simulink model "DriverSwRequest"  (R2023a)
settings: Solver=FixedStepDiscrete  StartTime=0.0  StopTime=10.0  FixedStep=0.01  RelTol=1e-3
undefined symbols (not defined in the file): reqMode
libraries: simulink x20
settings Model: RequirementInfo={} %GIDa_1a0f7f75_7b2a_416a_8409_7d146d7c864c  DataDictionary=crs_controllerdic.sldd  EnableAccessToBaseWorkspace=off  Creator=The MathWorks, Inc.  LastModifiedBy=shayashi
settings SolverCC: AlgebraicLoopSolver=TrustRegion
settings DataIOCC: SaveOutput=off  SignalLogging=off  DSMLogging=off  SaveTime=off  ReturnWorkspaceOutputs=off
settings OptimizationCC: DefaultParameterBehavior=Inlined  PassReuseOutputArgsAs=Individual arguments  EfficientTunableParamExpr=on
settings DebuggingCC: ParameterTunabilityLossMsg=error  UnconnectedInputMsg=warning  UnconnectedOutputMsg=warning  UnconnectedLineMsg=warning  ArithmeticOperatorsInVariantConditions=warning
settings ModelReferenceCC: EnableRefExpFcnMdlSchedulingChecks=on
settings SFSimCC: SimUseLocalCustomCode=off  CustomCodeUndefinedFunction=UseInterfaceOnly
settings RTWCC: Description=Embedded Coder  SystemTargetFile=ert.tlc  GenCodeOnly=on  TemplateMakefile=ert_default_tmf  GenerateReport=on  RTWUseLocalCustomCode=off  IncludeHyperlinkInReport=on  GenerateTraceInfo=on  GenerateTraceReport=on  GenerateTraceReportSl=on  GenerateTraceReportSf=on  GenerateTraceReportEml=on  DLArmComputeVersion=19.05
settings CodeAppCC: ForceParamTrailComments=on  IgnoreCustomStorageClasses=off  OperatorAnnotations=on  SimulinkDataObjDesc=on  SFDataObjDesc=on  MATLABFcnDesc=on  InsertBlockDesc=on  StateflowObjectComments=on  MATLABSourceComments=on  ReqsInCode=on
settings ERTTargetCC: TargetLangStandard=C99 (ISO)  GenerateSampleERTMain=on  InlinedParameterPlacement=NonHierarchical  ERTCustomFileTemplate=example_file_process.tlc

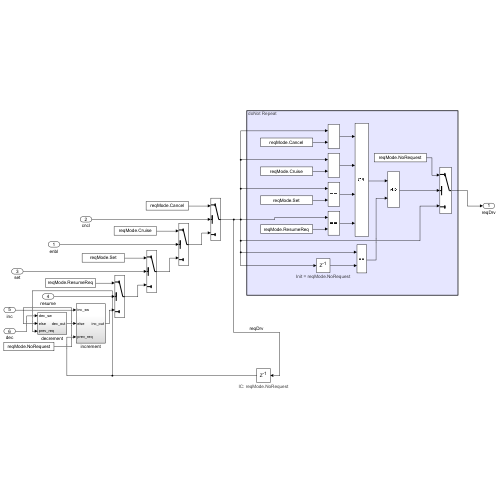
[thumbnail: Simulink's stored preview of the top-level diagram]
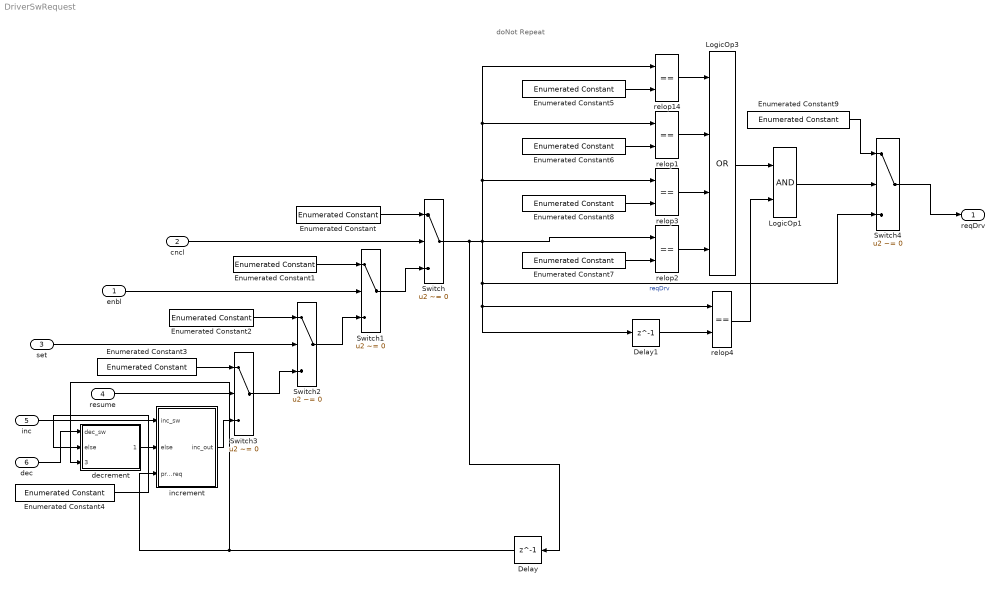
== system DriverSwRequest ==
  note: doNot Repeat
  enbl : Inport  RequirementInfo={} %GIDa_4508f6a0_e7ed_4c0c_b02f_e6c65ac58099  OutDataTypeStr=boolean  PortDimensions=1  SampleTime=[0.01,0]
  cncl : Inport  RequirementInfo={} %GIDa_777085d3_b4d2_4867_a99c_54d73e43353b  Port=2  OutDataTypeStr=boolean  PortDimensions=1  SampleTime=[0.01,0]
  set : Inport  RequirementInfo={} %GIDa_566ec4e5_1616_45a9_84b9_4b82093d43d0  Port=3  OutDataTypeStr=boolean  PortDimensions=1  SampleTime=[0.01,0]
  resume : Inport  RequirementInfo={} %GIDa_f47bc17c_749a_4107_a949_0eab582d2bca  Port=4  OutDataTypeStr=boolean  PortDimensions=1  SampleTime=[0.01,0]
  inc : Inport  RequirementInfo={} %GIDa_80e0c4b2_6973_4ccf_b5dd_c8c6037396b7  Port=5  OutDataTypeStr=boolean  PortDimensions=1  SampleTime=[0.01,0]
  dec : Inport  RequirementInfo={} %GIDa_10a9b33d_cc70_4197_af46_bb7a1e78c832  Port=6  OutDataTypeStr=boolean  PortDimensions=1  SampleTime=[0.01,0]
  Delay : Delay  RequirementInfo={} %GIDa_68175291_116a_4e9f_b16d_dc96f281223d  DelayLength=1  InitialCondition=reqMode.NoRequest
      settings: AttributesFormatString=IC: %<InitialCondition>
  Delay1 : Delay  RequirementInfo={} %GIDa_d6b95c2e_a65f_4493_8143_d1486d4778b4  DelayLength=1  InitialCondition=reqMode.NoRequest
      settings: AttributesFormatString=Init = %<InitialCondition>
  Enumerated Constant : simulink/Sources/Enumerated Constant  OutDataTypeStr=Enum: reqMode  Value=reqMode.Cancel  SampleTime=inf
  Enumerated Constant1 : simulink/Sources/Enumerated Constant  OutDataTypeStr=Enum: reqMode  Value=reqMode.Cruise  SampleTime=inf
  Enumerated Constant2 : simulink/Sources/Enumerated Constant  OutDataTypeStr=Enum: reqMode  Value=reqMode.Set  SampleTime=inf
  Enumerated Constant3 : simulink/Sources/Enumerated Constant  OutDataTypeStr=Enum: reqMode  Value=reqMode.ResumeReq  SampleTime=inf
  Enumerated Constant4 : simulink/Sources/Enumerated Constant  OutDataTypeStr=Enum: reqMode  Value=reqMode.NoRequest  SampleTime=inf
  Enumerated Constant5 : simulink/Sources/Enumerated Constant  RequirementInfo={} %GIDa_ef8ed732_da69_4c8b_bc64_a465f5b14abf  OutDataTypeStr=Enum: reqMode  Value=reqMode.Cancel  SampleTime=inf
  Enumerated Constant6 : simulink/Sources/Enumerated Constant  RequirementInfo={} %GIDa_c1772e6c_bb71_4ad8_975e_c7ee373e63bc  OutDataTypeStr=Enum: reqMode  Value=reqMode.Cruise  SampleTime=inf
  Enumerated Constant7 : simulink/Sources/Enumerated Constant  RequirementInfo={} %GIDa_f54ea5ac_ef42_4b75_8a76_95d17a0134f8  OutDataTypeStr=Enum: reqMode  Value=reqMode.ResumeReq  SampleTime=inf
  Enumerated Constant8 : simulink/Sources/Enumerated Constant  RequirementInfo={} %GIDa_112450ca_03fa_47b5_9a8a_ebc3c6421e0d  OutDataTypeStr=Enum: reqMode  Value=reqMode.Set  SampleTime=inf
  Enumerated Constant9 : simulink/Sources/Enumerated Constant  RequirementInfo={} %GIDa_23a28ec2_e6d1_434c_b80a_f07e608d4a03  OutDataTypeStr=Enum: reqMode  Value=reqMode.NoRequest  SampleTime=inf
  LogicOp1 : Logic  RequirementInfo={} %GIDa_ecd5b7bc_5d6b_4482_981e_50992a66f68b  AllPortsSameDT=off  OutDataTypeStr=boolean
  LogicOp3 : Logic  RequirementInfo={} %GIDa_ca94c19b_f51b_4b32_a882_c6d3a9962c39  Operator=OR  Inputs=4  AllPortsSameDT=off  OutDataTypeStr=boolean
  Switch : Switch  RequirementInfo={} %GIDa_046a32fa_7ae2_49ac_a43e_97d5ba4d0ef1  Criteria=u2 ~= 0  SaturateOnIntegerOverflow=off  InputSameDT=off
  Switch1 : Switch  RequirementInfo={} %GIDa_a26e3059_7a76_4e65_bcdd_c8d0ea685a20  Criteria=u2 ~= 0  SaturateOnIntegerOverflow=off  InputSameDT=off
  Switch2 : Switch  RequirementInfo={} %GIDa_68dec6e4_18d7_4e30_88c6_cf447ee8f5f1  Criteria=u2 ~= 0  SaturateOnIntegerOverflow=off  InputSameDT=off
  Switch3 : Switch  RequirementInfo={} %GIDa_c5846875_17c7_4c5a_a421_798f11c793cd  Criteria=u2 ~= 0  SaturateOnIntegerOverflow=off  InputSameDT=off
  Switch4 : Switch  RequirementInfo={} %GIDa_2debf59d_6a09_47fd_9563_b31545431772  Criteria=u2 ~= 0  SaturateOnIntegerOverflow=off  InputSameDT=off
  decrement : Subsystem  RequirementInfo={} %GIDa_b039651b_ad66_4ef3_8356_aef1393db1ab
  increment : Subsystem  RequirementInfo={} %GIDa_045c4eb9_abb8_473f_8004_b486deae16e4
  relop1 : RelationalOperator  RequirementInfo={} %GIDa_a3e85dc2_7475_4e31_a1ef_9117b650e758  Operator===  OutDataTypeStr=boolean  InputSameDT=off
  relop14 : RelationalOperator  RequirementInfo={} %GIDa_00c67d03_1f06_4643_ba21_636ebd7974bc  Operator===  OutDataTypeStr=boolean  InputSameDT=off
  relop2 : RelationalOperator  RequirementInfo={} %GIDa_3fe660c7_d5a0_4924_94c4_c620b0d879ab  Operator===  OutDataTypeStr=boolean  InputSameDT=off
  relop3 : RelationalOperator  RequirementInfo={} %GIDa_c1c6598f_eb24_416a_a01d_0895211c2c29  Operator===  OutDataTypeStr=boolean  InputSameDT=off
  relop4 : RelationalOperator  RequirementInfo={} %GIDa_064491b2_0235_49b5_a594_975ac74d463f  Operator===  OutDataTypeStr=boolean  InputSameDT=off
  reqDrv : Outport  RequirementInfo={} %GIDa_09f567f9_de75_4f5b_9ac7_ad71f062b6d3  OutDataTypeStr=Enum: reqMode  PortDimensions=1  SampleTime=[0.01,0]  VectorParamsAs1DForOutWhenUnconnected=off
  wires:
  Enumerated Constant/1 -> Switch/1
  Switch/1 -> Delay1/1, relop4/1, Switch4/3, relop1/1, relop14/1, relop3/1, relop2/1, Delay/1  "reqDrv"
  cncl/1 -> Switch/2
  Enumerated Constant1/1 -> Switch1/1
  Switch1/1 -> Switch/3
  set/1 -> Switch2/2
  Enumerated Constant2/1 -> Switch2/1
  resume/1 -> Switch3/2
  Enumerated Constant3/1 -> Switch3/1
  Switch3/1 -> Switch2/3
  Switch2/1 -> Switch1/3
  dec/1 -> decrement/1(dec_sw)
  Enumerated Constant4/1 -> decrement/2(else)
  inc/1 -> increment/1(inc_sw)
  decrement/1(dec_out) -> increment/2(else)
  increment/1(inc_out) -> Switch3/3
  Delay/1 -> decrement/3(prev_req), increment/3(prev_req)
  Switch4/1 -> reqDrv/1
  enbl/1 -> Switch1/2
  Enumerated Constant5/1 -> relop14/2
  Enumerated Constant6/1 -> relop1/2
  Enumerated Constant8/1 -> relop3/2
  Enumerated Constant7/1 -> relop2/2
  relop14/1 -> LogicOp3/1
  relop1/1 -> LogicOp3/2
  relop3/1 -> LogicOp3/3
  relop2/1 -> LogicOp3/4
  Delay1/1 -> relop4/2
  relop4/1 -> LogicOp1/2
  LogicOp3/1 -> LogicOp1/1
  LogicOp1/1 -> Switch4/2
  Enumerated Constant9/1 -> Switch4/1

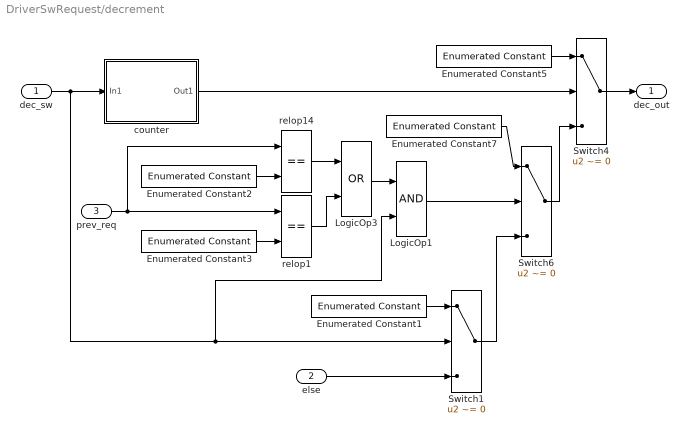
== system DriverSwRequest/decrement ==
  dec_sw : Inport  RequirementInfo={} %GIDa_e04a6fa3_5177_4f8f_83c2_e532fc2a23b3
  else : Inport  RequirementInfo={} %GIDa_8784e85d_910c_4d9c_b8e4_d1614a68b5de  Port=2
  prev_req : Inport  RequirementInfo={} %GIDa_1db7963f_fa03_4fcf_8601_ab653705e851  Port=3
  Enumerated Constant1 : simulink/Sources/Enumerated Constant  RequirementInfo={} %GIDa_e1739de0_be3b_4ad9_a7c8_e60b84ceb6dc  OutDataTypeStr=Enum: reqMode  Value=reqMode.Dec_Short  SampleTime=inf
  Enumerated Constant2 : simulink/Sources/Enumerated Constant  RequirementInfo={} %GIDa_2093fe57_fae4_4bcb_9d45_e1fa77b16bf7  OutDataTypeStr=Enum: reqMode  Value=reqMode.Dec_Short  SampleTime=inf
  Enumerated Constant3 : simulink/Sources/Enumerated Constant  RequirementInfo={} %GIDa_d51aa419_16a3_4011_8243_7bf457171348  OutDataTypeStr=Enum: reqMode  Value=reqMode.Dec_Middle  SampleTime=inf
  Enumerated Constant5 : simulink/Sources/Enumerated Constant  RequirementInfo={} %GIDa_7c8bfdb9_d495_4308_ba41_7ba38f3cde36  OutDataTypeStr=Enum: reqMode  Value=reqMode.Dec_Long  SampleTime=inf
  Enumerated Constant7 : simulink/Sources/Enumerated Constant  RequirementInfo={} %GIDa_6e38ca4f_a665_4587_98b7_59c945c883f0  OutDataTypeStr=Enum: reqMode  Value=reqMode.Dec_Middle  SampleTime=inf
  LogicOp1 : Logic  RequirementInfo={} %GIDa_19988df2_5924_4fe9_9b56_4b7e4a7ac21c  AllPortsSameDT=off  OutDataTypeStr=boolean
  LogicOp3 : Logic  RequirementInfo={} %GIDa_c6b2bd35_9314_432c_a51f_a995ada239d9  Operator=OR  AllPortsSameDT=off  OutDataTypeStr=boolean
  Switch1 : Switch  RequirementInfo={} %GIDa_9a1e8653_20ee_437d_b4d2_9eade4c7e0d0  Criteria=u2 ~= 0  SaturateOnIntegerOverflow=off  InputSameDT=off
  Switch4 : Switch  RequirementInfo={} %GIDa_29c33e47_8a99_43a9_b4d7_9dfafa8ec43c  Criteria=u2 ~= 0  SaturateOnIntegerOverflow=off  InputSameDT=off
  Switch6 : Switch  RequirementInfo={} %GIDa_417537e7_4cad_4653_8680_5824e2aabc5c  Criteria=u2 ~= 0  SaturateOnIntegerOverflow=off  InputSameDT=off
  counter : Subsystem  RequirementInfo={} %GIDa_44ecd491_48ea_46f1_a719_8962cb923bfb  DisableCoverage=on  mask(SLDV counter){CountValue=50, OutDataTypeStr=uint8}
      mask prompts: CountValue "Count value"; OutDataTypeStr "Data type"
      mask help: A counter block optimized for Simulink Design Verifier test case generation. If the input is true for consecutive steps which is specified the Count value parameter, then the output is TRUE, otherwise it is FALSE.
      mask init:
      | if CountValue < 0 || CountValue > intmax(OutDataTypeStr)
      |     error('Specified count value needs to be within 0-%d.',intmax(OutDataTypeStr))
      | end
      mask Display: disp(sprintf('Counter (%s)\nCount:%d',OutDataTypeStr,CountValue))
  relop1 : RelationalOperator  RequirementInfo={} %GIDa_ec26ee53_bcc4_4ba6_8801_88fb03838afa  Operator===  OutDataTypeStr=boolean  InputSameDT=off
  relop14 : RelationalOperator  RequirementInfo={} %GIDa_257543b3_eee1_4269_bc05_e267b3f99015  Operator===  OutDataTypeStr=boolean  InputSameDT=off
  dec_out : Outport  RequirementInfo={} %GIDa_127bbb26_1727_4374_89f9_07c640846242  VectorParamsAs1DForOutWhenUnconnected=off
  wires:
  LogicOp1/1 -> Switch6/2
  LogicOp3/1 -> LogicOp1/1
  relop1/1 -> LogicOp3/2
  relop14/1 -> LogicOp3/1
  prev_req/1 -> relop1/1, relop14/1
  Enumerated Constant3/1 -> relop1/2
  Enumerated Constant2/1 -> relop14/2
  Enumerated Constant1/1 -> Switch1/1
  else/1 -> Switch1/3
  dec_sw/1 -> Switch1/2, LogicOp1/2, counter/1(In1)
  Switch1/1 -> Switch6/3
  counter/1(Out1) -> Switch4/2
  Switch6/1 -> Switch4/3
  Enumerated Constant7/1 -> Switch6/1
  Switch4/1 -> dec_out/1
  Enumerated Constant5/1 -> Switch4/1

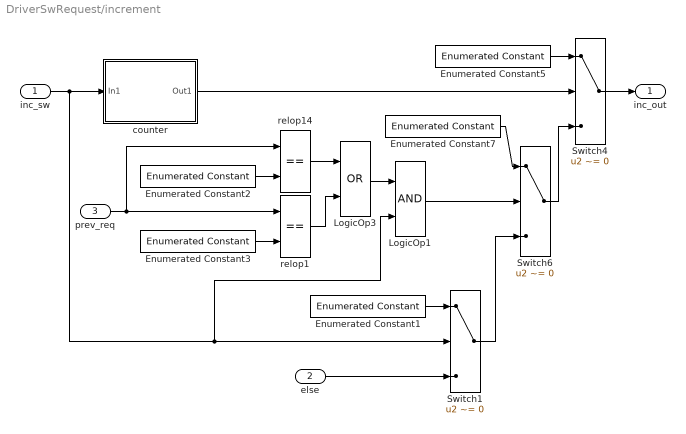
== system DriverSwRequest/increment ==
  inc_sw : Inport  RequirementInfo={} %GIDa_eafef2e8_8427_4ff8_bae9_6965afacd1cc
  else : Inport  RequirementInfo={} %GIDa_f47e1157_5432_4339_82ce_b948fad1a93a  Port=2
  prev_req : Inport  RequirementInfo={} %GIDa_27b9c7b3_1080_4a97_9064_8e9a7ec4f4cc  Port=3
  Enumerated Constant1 : simulink/Sources/Enumerated Constant  RequirementInfo={} %GIDa_cdda409d_23a5_402f_86c5_cf29439bcb14  OutDataTypeStr=Enum: reqMode  Value=reqMode.Inc_Short  SampleTime=inf
  Enumerated Constant2 : simulink/Sources/Enumerated Constant  RequirementInfo={} %GIDa_b491db74_7231_4b12_91d9_81b14678a118  OutDataTypeStr=Enum: reqMode  Value=reqMode.Inc_Short  SampleTime=inf
  Enumerated Constant3 : simulink/Sources/Enumerated Constant  RequirementInfo={} %GIDa_8996fdc1_3f97_4d5a_8a9c_f829de38b95d  OutDataTypeStr=Enum: reqMode  Value=reqMode.Inc_Middle  SampleTime=inf
  Enumerated Constant5 : simulink/Sources/Enumerated Constant  RequirementInfo={} %GIDa_69556d18_13ca_44a3_9083_137d94a87bb4  OutDataTypeStr=Enum: reqMode  Value=reqMode.Inc_Long  SampleTime=inf
  Enumerated Constant7 : simulink/Sources/Enumerated Constant  RequirementInfo={} %GIDa_5193a7a6_7f6c_4b0f_a7c0_8219d089208e  OutDataTypeStr=Enum: reqMode  Value=reqMode.Inc_Middle  SampleTime=inf
  LogicOp1 : Logic  RequirementInfo={} %GIDa_33a3cc30_a365_48eb_bec6_c8857d7a6ed4  AllPortsSameDT=off  OutDataTypeStr=boolean
  LogicOp3 : Logic  RequirementInfo={} %GIDa_ca8612e9_cbbf_43a3_9d44_d736bfc808a1  Operator=OR  AllPortsSameDT=off  OutDataTypeStr=boolean
  Switch1 : Switch  RequirementInfo={} %GIDa_e458111a_1bee_4987_b412_cee89ae05192  Criteria=u2 ~= 0  SaturateOnIntegerOverflow=off  InputSameDT=off
  Switch4 : Switch  RequirementInfo={} %GIDa_8fa887ee_537a_4244_849f_ab3d451afe00  Criteria=u2 ~= 0  SaturateOnIntegerOverflow=off  InputSameDT=off
  Switch6 : Switch  RequirementInfo={} %GIDa_745fd177_d958_45f5_a334_1652316e59c3  Criteria=u2 ~= 0  SaturateOnIntegerOverflow=off  InputSameDT=off
  counter : Subsystem  RequirementInfo={} %GIDa_643bfb40_00f6_4403_8ae3_e854d175fe11  DisableCoverage=on  mask(SLDV counter){CountValue=50, OutDataTypeStr=uint8}
      mask prompts: CountValue "Count value"; OutDataTypeStr "Data type"
      mask help: A counter block optimized for Simulink Design Verifier test case generation. If the input is true for consecutive steps which is specified the Count value parameter, then the output is TRUE, otherwise it is FALSE.
      mask init:
      | if CountValue < 0 || CountValue > intmax(OutDataTypeStr)
      |     error('Specified count value needs to be within 0-%d.',intmax(OutDataTypeStr))
      | end
      mask Display: disp(sprintf('Counter (%s)\nCount:%d',OutDataTypeStr,CountValue))
  relop1 : RelationalOperator  RequirementInfo={} %GIDa_32202e1f_5904_4f7b_8e8e_4e8b72f08ac1  Operator===  OutDataTypeStr=boolean  InputSameDT=off
  relop14 : RelationalOperator  RequirementInfo={} %GIDa_70d1185d_960e_4b17_ad0d_404c89053196  Operator===  OutDataTypeStr=boolean  InputSameDT=off
  inc_out : Outport  RequirementInfo={} %GIDa_ca8e9415_6c9b_4c20_a936_d083468b689c  VectorParamsAs1DForOutWhenUnconnected=off
  wires:
  LogicOp1/1 -> Switch6/2
  LogicOp3/1 -> LogicOp1/1
  relop1/1 -> LogicOp3/2
  relop14/1 -> LogicOp3/1
  prev_req/1 -> relop1/1, relop14/1
  Enumerated Constant3/1 -> relop1/2
  Enumerated Constant2/1 -> relop14/2
  Enumerated Constant1/1 -> Switch1/1
  else/1 -> Switch1/3
  inc_sw/1 -> Switch1/2, LogicOp1/2, counter/1(In1)
  Switch1/1 -> Switch6/3
  counter/1(Out1) -> Switch4/2
  Switch6/1 -> Switch4/3
  Enumerated Constant7/1 -> Switch6/1
  Switch4/1 -> inc_out/1
  Enumerated Constant5/1 -> Switch4/1

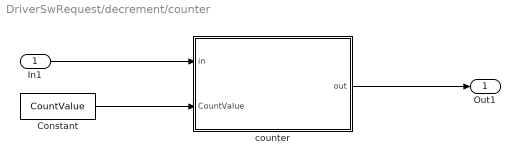
== system DriverSwRequest/decrement/counter ==
  In1 : Inport  RequirementInfo={} %GIDa_e8895a6b_5370_4bef_8bab_ba2870cc6e4c
  Constant : Constant  RequirementInfo={} %GIDa_1ce17d01_953a_4593_b594_5b0b83cc1cf7  Value=CountValue  OutDataTypeStr=OutDataTypeStr
  counter : MATLAB Function  RequirementInfo={} %GIDa_1ac197a8_f052_429a_bf44_539be74bf37e  TreatAsAtomicUnit=on
  Out1 : Outport  RequirementInfo={} %GIDa_7b79b25a_bdd1_4bd8_938e_441798da4365  VectorParamsAs1DForOutWhenUnconnected=off
  wires:
  In1/1 -> counter/1(in)
  counter/1(out) -> Out1/1
  Constant/1 -> counter/2(CountValue)

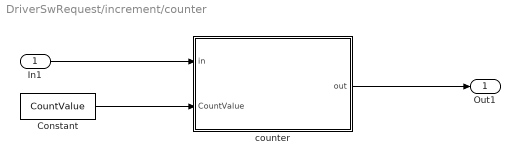
== system DriverSwRequest/increment/counter ==
  In1 : Inport  RequirementInfo={} %GIDa_7e7cd906_0c88_4135_af53_7298618ebc25
  Constant : Constant  RequirementInfo={} %GIDa_e6daeba8_b84d_4e7c_9a6e_f1f3f60fd2bc  Value=CountValue  OutDataTypeStr=OutDataTypeStr
  counter : MATLAB Function  RequirementInfo={} %GIDa_2a5db1d8_56ee_4145_9735_821485e00fe3  TreatAsAtomicUnit=on
  Out1 : Outport  RequirementInfo={} %GIDa_d295e170_73d6_4c14_b3c4_be5474d20575  VectorParamsAs1DForOutWhenUnconnected=off
  wires:
  In1/1 -> counter/1(in)
  counter/1(out) -> Out1/1
  Constant/1 -> counter/2(CountValue)

== matlab function DriverSwRequest/increment/counter/counter ==
  data: in input boolean size=1; out output boolean size=1; CountValue input uint8 size=1
function out = counter(in,CountValue)
%#codegen

persistent cnt;

% initialize
if isempty(cnt)
    cnt = cast(0,'like',CountValue);
end

% if enabled
if in
    % Output true if CountValue is reached
    if cnt >= CountValue
        out = true;
    else
        % Continue counting up and output false
        cnt = cnt + cast(1,'like',CountValue);
        out = false;
    end
else
    % if disabled, output false and reset
    cnt = cast(0,'like',CountValue);
    out = false;
end

== matlab function DriverSwRequest/decrement/counter/counter ==
  data: in input boolean size=1; out output boolean size=1; CountValue input uint8 size=1
function out = counter(in,CountValue)
%#codegen

persistent cnt;

% initialize
if isempty(cnt)
    cnt = cast(0,'like',CountValue);
end

% if enabled
if in
    % Output true if CountValue is reached
    if cnt >= CountValue
        out = true;
    else
        % Continue counting and output false        
        cnt = cnt + cast(1,'like',CountValue);
        out = false;
    end
else
    % if disabled, output false and reset
    cnt = cast(0,'like',CountValue);
    out = false;
end
